simulink model "DeadbeatStateSpace"  (R2016b)
settings: Solver=VariableStepAuto  StartTime=0.0  StopTime=10.0  RelTol=1e-3
values from neighbouring files (symbols this model uses):
  P = 1/s/(s+1)    [DeadbeatDesignerSS.m]
libraries: cstblocks x2
settings Model: Creator=capn  LastModifiedBy=capn

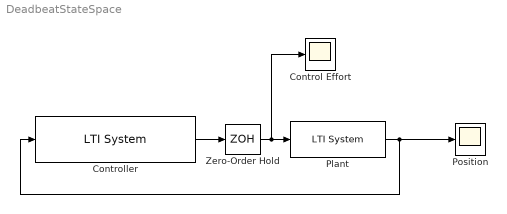
== system DeadbeatStateSpace ==
  Control Effort : Scope
  Controller : cstblocks/LTI System  sys=Cc  IC=[]
  Plant : cstblocks/LTI System  sys=ss(P)  IC=x0
  Position : Scope
  Zero-Order Hold : ZeroOrderHold  SampleTime=-1
  wires:
  Controller/1 -> Zero-Order Hold/1
  Zero-Order Hold/1 -> Control Effort/1, Plant/1
  Plant/1 -> Controller/1, Position/1
